simulink model "testEmplanner_cs_referencelinev01"  (R2021b)
settings: Solver=ode5  StartTime=0.0  StopTime=150  FixedStep=1/1000  RelTol=1e-3
PreLoadFcn:
  | mbxruntime.callbacks.PreLoadFcn(bdroot);
PostLoadFcn:
  | mbxruntime.callbacks.PostLoadFcn(bdroot);
InitFcn:
  | mbxruntime.callbacks.InitFcn(bdroot);
StartFcn:
  | mbxruntime.callbacks.StartFcn(bdroot);
StopFcn:
  | mbxruntime.callbacks.StopFcn(bdroot);
model workspace (MAT data in the model file):
  mbox_table : object (value not decoded)
  model_closed = 0
  sim_status = 0
values from neighbouring files (symbols this model uses):
  c_factor = 43.75    [emplanner_init.m]
  cf = -175016    [emplanner_init.m]
  cr = -130634    [emplanner_init.m]
  global_path_x = [-1.1448 -0.145417744933 0.852705365581 1.84955224935 2.84511712279 3.83939835808 4.83239585569 5.82411007764 6.81454169183 7.80369144113 8.79156009523 9.77814843293 ... (3001 elements, 3001x1)]    [global_path.mat]
  global_path_y = [14.6488 14.6488 14.6488 14.6488 14.6488 14.6488 14.6488 14.6488 14.6488 14.6488 14.6488 14.6488 ... (3001 elements, 3001x1)]    [global_path.mat]
  KD_PID_distance = 0.0    (= 0)    [emplanner_init.m]
  KD_PID_speed = 0    [emplanner_init.m]
  KI_PID_distance = 0.0    (= 0)    [emplanner_init.m]
  KI_PID_speed = 0    [emplanner_init.m]
  KP_PID_distance = 0.5    [emplanner_init.m]
  KP_PID_speed = 1.8    [emplanner_init.m]
  la = 1.265    [emplanner_init.m]
  lb = 2.947-1.265    (= 1.682)    [emplanner_init.m]
  LQR_K1 = k(:,1)'    [emplanner_init.m]
  LQR_K2 = k(:,2)'    [emplanner_init.m]
  LQR_K3 = k(:,3)'    [emplanner_init.m]
  LQR_K4 = k(:,4)'    [emplanner_init.m]
  m = 2020    [emplanner_init.m]
  rack_displacement = [-39.14 , -37.2 , -35.29 , -33.43 , -31.6 , -29.81 , -28.06 , -26.34 , -24.66 ,      -23.01 , -21.38 , -19.79 , -18.23 , -16.69 , -15.18 , -13.7 , -12.23 , -10.8 , -9.38 , -7.98 ,     -6.61 , -5.25 , -3.91 , -2.59 , -1.29 , 0 , 1.27 , 2.54 , 3.78 , 5.02 , 6.24 , 7.46 , 8.66 ,      9.86 , 11.05 , 12.24 , 13.41 , 14.59 , 15.76 , 16.92 , 18.09 , 19.25 , 20.42 , 21.59 , 22.76 ,      23.93 , 25.11 , 26 ...(+26 chars)    [emplanner_init.m]
  right_wheel_ground = [-70 ,-67.2 , -64.4 , -61.6 , -58.8 , -56 , -53.2 , -50.4 , -47.6 , -44.8 , -42 ,      -39.2 , -36.4 , -33.6 , -30.8 , -28 , -25.2 , -22.4 , -19.6 , -16.8 , -14 , -11.2 , -8.4 , -5.6 ,      -2.8 , 0 , 2.8 , 5.6 , 8.4 , 11.2 , 14 , 16.8 , 19.6 , 22.4 , 25.2 , 28 , 30.8 , 33.6 , 36.4 ,      39.2 , 42 , 44.8 , 47.6 , 50.4 , 53.2 , 56 , 58.8 , 61.6 , 64.4 , 67.2 , 70 ]    [emplanner_init.m]
  vx_break_point = zeros(1,5000)    [emplanner_init.m]
undefined symbols (not defined in the file or in its folder): aubr, DiscIntNeverNeededParam, tablebr, vubr, warningInitialVelocity, x0
libraries: simulink x19, PreScanSimulinkLibrary x9, simulink_extras x6, Solver_SF x1
(part 5 of 5)

== system testEmplanner_cs_referencelinev01/Audi_A8_Sedan_2/Dynamics_Simple/Chassis/Bicycle_model_[XYZ]/Z, Pitch_Motion & Roll_Motion/Configurable Subsystem1 ==
  In1 : Inport
  Integrator : Integrator
  Out1 : Outport
  wires:
  In1/1 -> Integrator/1
  Integrator/1 -> Out1/1

== system testEmplanner_cs_referencelinev01/Audi_A8_Sedan_2/Dynamics_Simple/Chassis/Bicycle_model_[XYZ]/Z, Pitch_Motion & Roll_Motion/Configurable Subsystem2 ==
  In1 : Inport
  Integrator : Integrator
  Out1 : Outport
  wires:
  In1/1 -> Integrator/1
  Integrator/1 -> Out1/1

== system testEmplanner_cs_referencelinev01/Audi_A8_Sedan_2/Dynamics_Simple/Chassis/Bicycle_model_[XYZ]/Z, Pitch_Motion & Roll_Motion/Configurable Subsystem3 ==
  In1 : Inport
  Integrator : Integrator
  Out1 : Outport
  wires:
  In1/1 -> Integrator/1
  Integrator/1 -> Out1/1

== system testEmplanner_cs_referencelinev01/Audi_A8_Sedan_2/Dynamics_Simple/Chassis/Bicycle_model_[XYZ]/Z, Pitch_Motion & Roll_Motion/Configurable Subsystem4 ==
  In1 : Inport
  Integrator : Integrator
  Out1 : Outport
  wires:
  In1/1 -> Integrator/1
  Integrator/1 -> Out1/1

== system testEmplanner_cs_referencelinev01/Audi_A8_Sedan_2/Dynamics_Simple/Chassis/Bicycle_model_[XYZ]/Z, Pitch_Motion & Roll_Motion/Configurable Subsystem5 ==
  In1 : Inport
  Integrator : Integrator
  Out1 : Outport
  wires:
  In1/1 -> Integrator/1
  Integrator/1 -> Out1/1

== system testEmplanner_cs_referencelinev01/Audi_A8_Sedan_2/Dynamics_Simple/Chassis/Bicycle_model_[XYZ]/Z, Pitch_Motion & Roll_Motion/Configurable Subsystem9 ==
  In1 : Inport
  Derivative : Derivative
  Out1 : Outport
  wires:
  In1/1 -> Derivative/1
  Derivative/1 -> Out1/1

== system testEmplanner_cs_referencelinev01/Audi_A8_Sedan_2/Dynamics_Simple/Chassis/FrontTyre/AlphaFront/Enabled Subsystem ==
  In : Inport
  Enable : EnablePort  PropagateVarSize=During execution
  AlphaFront : Fcn  Expr=-atan( (u(2)+u(3)*p.a)/u(1) )
  Alpha : Outport  OutputWhenDisabled=reset  InitialOutput=[0]
  wires:
  AlphaFront/1 -> Alpha/1
  In/1 -> AlphaFront/1

== system testEmplanner_cs_referencelinev01/Audi_A8_Sedan_2/Dynamics_Simple/Chassis/RearTyre/AlphaRear/Enabled Subsystem ==
  In : Inport
  Enable : EnablePort  PropagateVarSize=During execution
  AlphaRear : Fcn  Expr=-atan( (u(2)-u(3)*p.b)/u(1) )
  Alpha : Outport  OutputWhenDisabled=reset  InitialOutput=[0]
  wires:
  AlphaRear/1 -> Alpha/1
  In/1 -> AlphaRear/1

== system testEmplanner_cs_referencelinev01/Audi_A8_Sedan_2/Trajectories/Traj2State1/Traj2State2/Traj2MuxState_Ext/demux ==
  traj : Inport
  Demux : Demux  Outputs=18
  x : Outport
  y : Outport  Port=2
  z : Outport  Port=3
  velx : Outport  Port=4
  vely : Outport  Port=5
  velz : Outport  Port=6
  R : Outport  Port=7
  P : Outport  Port=8
  Y : Outport  Port=9
  velR : Outport  Port=10
  velP : Outport  Port=11
  velY : Outport  Port=12
  accx : Outport  Port=13
  accy : Outport  Port=14
  accz : Outport  Port=15
  accR : Outport  Port=16
  accP : Outport  Port=17
  accY : Outport  Port=18
  wires:
  Demux/18 -> accY/1
  Demux/17 -> accP/1
  Demux/16 -> accR/1
  Demux/15 -> accz/1
  Demux/14 -> accy/1
  Demux/13 -> accx/1
  Demux/12 -> velY/1
  Demux/11 -> velP/1
  Demux/10 -> velR/1
  Demux/9 -> velz/1
  Demux/8 -> vely/1
  Demux/7 -> velx/1
  Demux/6 -> Y/1
  Demux/5 -> P/1
  traj/1 -> Demux/1
  Demux/4 -> R/1
  Demux/3 -> z/1
  Demux/2 -> y/1
  Demux/1 -> x/1

== system testEmplanner_cs_referencelinev01/Audi_A8_Sedan_2/Dynamics_Simple/Chassis/Bicycle_model_[XYZ]/X_Motion/Max RPM and zero- velocity detection/Configurable Subsystem ==
  Step : Step  Time=0.0001  Before=1  After=0  SampleTime=0
  Out1 : Outport
  wires:
  Step/1 -> Out1/1

== system testEmplanner_cs_referencelinev01/Audi_A8_Sedan_2/Dynamics_Simple/Chassis/Bicycle_model_[XYZ]/X_Motion/Max RPM and zero- velocity detection/SR-Memory ==
  Signal : Inport
  Set : Inport  Port=2
  Reset : Inport  Port=3
  Constant : Constant  Value=0
  Detect Rise Positive : simulink/Logic and Bit Operations/Detect Rise Positive  vinit=0  OutDataTypeStr=uint8
  Detect Rise Positive1 : simulink/Logic and Bit Operations/Detect Rise Positive  vinit=0  OutDataTypeStr=uint8
  Manual Switch : ManualSwitch
  Manual Switch1 : ManualSwitch
  Switch : Switch  Criteria=u2 ~= 0
  Switch1 : Switch  Criteria=u2 ~= 0
  Unit Delay : UnitDelay  SampleTime=-1  HasFrameUpgradeWarning=on
  Out : Outport
  wires:
  Constant/1 -> Switch1/1
  Switch/1 -> Switch1/3
  Switch1/1 -> Unit Delay/1, Out/1
  Manual Switch1/1 -> Switch1/2
  Reset/1 -> Manual Switch1/2, Detect Rise Positive1/1
  Detect Rise Positive1/1 -> Manual Switch1/1
  Signal/1 -> Switch/1
  Unit Delay/1 -> Switch/3
  Set/1 -> Detect Rise Positive/1, Manual Switch/2
  Detect Rise Positive/1 -> Manual Switch/1
  Manual Switch/1 -> Switch/2

== matlab function testEmplanner_cs_referencelinev01/Audi_A8_Sedan_1/decision&planning module/referenceline provider/MATLAB Function ==
  data: x_set input; match_point_index_set output; y_set input; frenet_path_x input; frenet_path_y input; frenet_path_heading input; frenet_path_kappa input; proj_x_set output; proj_y_set output; proj_heading_set output; proj_kappa_set output
function [match_point_index_set,proj_x_set,proj_y_set,proj_heading_set,proj_kappa_set] = ...
	fcn(x_set,y_set,frenet_path_x,frenet_path_y,frenet_path_heading,frenet_path_kappa)
	
%该函数将批量计算x_set,y_set中(x,y) 在frenet坐标系下的投影信息
%输入： x_set，y_set 待投影的点的集合
	%x_set,y_set,frenet_path_x,frenet_path_y,frenet_path_heading,frenet_path_kappa
	%曲线在直角坐标系下的x,y,heading,kappa
%输出：math_point_index_set 匹配点在frenet_path下的编号的集合（即从全局路径的第一个点开始数，第几个点是匹配点）

%由于事先不知道x_set中有多少个点需要投影，因此事先声明一个最大数量的点作为缓冲

n = 128;
%并且不知道投影点的数量，所以也不知道输出的数量，因此输出也要做缓冲，用nan表示不存在的点
%初始化输出最多为128个点。
%输出初始化
match_point_index_set = ones(n,1) * nan;
proj_x_set = ones(n,1) * nan;
proj_y_set = ones(n,1) * nan;
proj_heading_set = ones(n,1) * nan;
proj_kappa_set = ones(n,1) * nan;

%找匹配点，需要利用上一个周期的结果作为下一个周期遍历的起点，因此需要声明两个全局变量
persistent is_first_run;
persistent pre_match_point_index_set;
persistent pre_frenet_path_x;
persistent pre_frenet_path_y;
persistent pre_frenet_path_heading;
persistent pre_frenet_path_kappa;

%算法主函数入口

if isempty(is_first_run)
	% 该if分支表示函数首次运行
	is_first_run = 0; %赋值
	pre_frenet_path_x = frenet_path_x;
	pre_frenet_path_y = frenet_path_y;
	pre_frenet_path_heading = frenet_path_heading;
	pre_frenet_path_kappa = frenet_path_kappa;
	%记录首次运行计算的匹配点的结果供下个周期运行，先初始化
	pre_match_point_index_set = ones(n,1) * nan;
	
	%对x_set,y_set的点做遍历，找到他们的匹配点
	for i = 1 : length(x_set)
		%首次运行时，没有任何提示，只能从frenet_path的第一个点开始找
		start_search_index = 1;
		%声明increa_count,用于表示在遍历时distance连续增大的次数
		increase_count = 0;
		%开始遍历
		min_distance = inf;
		for j = start_search_index : length(frenet_path_x)
			distance = (x_set(i) - frenet_path_x(j))^2 + (y_set(i) - frenet_path_y(j))^2;
			%处理最小值
			if distance < min_distance
				min_distance = distance;
				match_point_index_set(i) = j; %math_point_index_set存放匹配点的序号
				increase_count = 0;
			else
				increase_count = increase_count + 1;
			end
			% 如果连续distanc增加50次,就不要再遍历了，节省时间
			if increase_count > 50 
				break;
			end	
		end
		%如何通过匹配点计算投影点，参考《自动驾驾驶控制算法第七讲》
		%或者《自动驾驶决策规划算法》第一章第三节
		
		%取出匹配点的编号
		match_point_index = match_point_index_set(i);
		
		%取出匹配点信息
		match_point_x = frenet_path_x(match_point_index);
		match_point_y = frenet_path_y(match_point_index);
		match_point_heading = frenet_path_heading(match_point_index);
		match_point_kappa = frenet_path_kappa(match_point_index);
		
		% 计算匹配点的位置向量和方向向量
		vector_match_point = [match_point_x;match_point_y];%位置向量
		vector_match_point_direction = [cos(match_point_heading);sin(match_point_heading)];%方向向量，全局坐标系下（大地坐标系）
		
		%声明待投影点的位矢
		vector_r = [x_set(i);y_set(i)];
		
		%通过匹配点计算投影点
		vector_d = vector_r - vector_match_point;
		ds = vector_d' * vector_match_point_direction;
		vector_proj_point = vector_match_point + vector_match_point_direction *ds;
		proj_heading = match_point_heading + match_point_kappa * ds;
		proj_kappa = match_point_kappa;
		
		%计算结果输出 
		proj_x_set(i) = vector_proj_point(1);
		proj_y_set(i) = vector_proj_point(2);
		proj_heading_set(i) = proj_heading;
		proj_kappa_set(i) = proj_kappa;
	end
	
	%匹配点的计算结果保存，供下一个周期使用
	pre_match_point_index_set = match_point_index_set;
else
	% 此分支不是首次运行
	
	%对每个x_set上的点做处理
	for i = 1 : length(x_set)
		%不是首次运行，对于点x_set(i),y_set(i)来说，start_search_index = pre_match_point_index_set(i)
		start_search_index = pre_match_point_index_set(i);%上个周期匹配点的编号作为本周期搜索的起点
		
		%声明increa_count,用于表示在遍历时distance连续增大的次数
		increase_count = 0;
		%开始遍历
		
		%这里多了一个步骤，判断遍历的方向
		%计算上个周期匹配点的位失
		vector_pre_match_point = [pre_frenet_path_x(start_search_index); pre_frenet_path_y(start_search_index)];
		vector_pre_match_point_direction = ...
			[cos(pre_frenet_path_heading(start_search_index));sin(pre_frenet_path_heading(start_search_index))];
		
		% 判断遍历的方向
		flag = ([x_set(i);y_set(i)] - vector_pre_match_point)' * vector_pre_match_point_direction;
		
		min_distance = inf;
		
		if flag > 0.001 
			for j = start_search_index : length(frenet_path_x)
				distance = (x_set(i) - frenet_path_x(j))^2 + (y_set(i) - frenet_path_y(j))^2;
				%处理最小值
				if distance < min_distance
					min_distance = distance;
					match_point_index_set(i) = j; %math_point_index_set存放匹配点的序号
					increase_count = 0;
				else
					increase_count = increase_count + 1;
				end
				% 如果连续distanc增加5次,就不要再遍历了，节省时间
				if increase_count > 5 
					break;
				end
			end
		elseif flag < -0.001
			for j = start_search_index :-1: 1
				distance = (x_set(i) - frenet_path_x(j))^2 + (y_set(i) - frenet_path_y(j))^2;
				%处理最小值
				if distance < min_distance
					min_distance = distance;
					match_point_index_set(i) = j; %math_point_index_set存放匹配点的序号
					increase_count = 0;
				else
					increase_count = increase_count + 1;
				end
				% 如果连续distanc增加50次,就不要再遍历了，节省时间
				if increase_count > 5 
					break;
				end
			end
		else
			match_point_index_set(i) = start_search_index;
		end
			
		%如何通过匹配点计算投影点，参考《自动驾驾驶控制算法第七讲》
		%或者《自动驾驶决策规划算法》第一章第三节
		
		%取出匹配点的编号
		match_point_index = match_point_index_set(i);
		
		%取出匹配点信息
		match_point_x = frenet_path_x(match_point_index);
		match_point_y = frenet_path_y(match_point_index);
		match_point_heading = frenet_path_heading(match_point_index);
		match_point_kappa = frenet_path_kappa(match_point_index);
		
		% 计算匹配点的位置向量和方向向量
		vector_match_point = [match_point_x;match_point_y];%位置向量
		vector_match_point_direction = [cos(match_point_heading);sin(match_point_heading)];%方向向量
		
		%声明待投影点的位矢
		vector_r = [x_set(i);y_set(i)];
		
		%通过匹配点计算投影点
		vector_d = vector_r - vector_match_point;
		ds = vector_d' * vector_match_point_direction;
		vector_proj_point = vector_match_point + ds * vector_match_point_direction;
		proj_heading = match_point_heading + match_point_kappa * ds;
		proj_kappa = match_point_kappa;
		
		%计算结果输出 
		proj_x_set(i) = vector_proj_point(1);
		proj_y_set(i) = vector_proj_point(2);
		proj_heading_set(i) = proj_heading;
		proj_kappa_set(i) = proj_kappa;
	end
	
	%匹配点的计算结果保存，供下一个周期使用
	pre_match_point_index_set = match_point_index_set;
	pre_frenet_path_x = frenet_path_x;
	pre_frenet_path_y = frenet_path_y;
	pre_frenet_path_heading = frenet_path_heading;
	pre_frenet_path_kappa = frenet_path_kappa;
end

== matlab function testEmplanner_cs_referencelinev01/Audi_A8_Sedan_1/decision&planning module/referenceline provider/MATLAB Function1 ==
  data: path_x input; path_heading output; path_y input; path_kappa output
function [path_heading,path_kappa] = fcn(path_x,path_y)
%该函数将计算path的切线方向与x轴的夹角和曲率
%输入：path_x,path_y路径的坐标（全局坐标系下）
%输出：path_heading,path_kappa 路径的heading和曲率
%原理：heading = arctan(dy/dx)
%  kappa = dheading /ds
%  ds = (dx^2 + dy^2)^0.5


%注意，角度的多值性会带来很大的麻烦，需要慎重处理
%例如： x与 x+2*pi代表同一个角度，这种多值性在曲率计算的时候会带来麻烦
%比如： 原本是（0.1 -（-0.1））/ ds,但是如果计算出得-0.1多了一个2*pi
%kappa 就等于(0.1 -(-0.1 + 2*pi)) /ds 曲率就会变得非常大
%还有若采用中点欧拉法计算heading时，即使用 (y2 - y1) / (x2 - x1)的反正切计算一个角度，用(y1 - y0)/(x1 - x0)的反正切
%又计算了一个角度，然后加起来除以2，如果精确值是(a1 + a2)/2,但是最终计算结果可能是(a1 + a2 + 2pi) / 2
%还有tan(x) = tan(x + pi） 所以 arctan(tan(x)) 可能等于x,也可能等于x + pi
%角度的处理非常麻烦，而且角度处理不当往往是许多奇怪错误的源头
%

dx = diff(path_x);
dy = diff(path_y);%计算差分

%用中点欧拉法要比向前欧拉法和向后欧拉法要更精确，但是也可能计算出的结果比精确值多一个pi
%在这里对dx,dy做中点欧拉法，使用四象限反正切计算角度

dx_pre = [dx(1);dx];
dx_after = [dx;dx(end)];
dx_final = (dx_pre + dx_after) / 2;

dy_pre = [dy(1);dy];
dy_after = [dy;dy(end)];
dy_final = (dy_pre + dy_after) / 2;

ds_final = sqrt(dx_final.^2 + dy_final.^2);
path_heading = atan2(dy_final,dx_final);

%atan2(b，a)：4象限反正切，

%　　　　计算b/a对应的反正切值，求点(a，b)对应的角
% 　　　　　(a，b)位于第一象限时，atan2(b，a)取值  0 ~ pi/2
% 　　　　　(a，b)位于第二象限时，atan2(b，a)取值  pi/2 ~ pi
% 　　　　　(a，b)位于第三象限时，atan2(b，a)取值   -pi ~ -pi/2
% 　　　　　(a，b)位于第四象限时，atan2(b，a)取值   -pi/2 ~ 0
%

%中点欧拉法
dheading = diff(path_heading);%差分，size变成length(path_heading) - 1
dheading_pre = [dheading(1);dheading]; %插入一个首元素
dheading_after = [dheading;dheading(end)]; %插入一个尾元素
dheading_final = (dheading_pre + dheading_after) / 2;
%为了防止dheading出现一个2*pi的错误，假设真实的heading较小，用sin(dheading)近似dheading
path_kappa = sin(dheading_final)./ds_final;

== matlab function testEmplanner_cs_referencelinev01/Audi_A8_Sedan_2/PathFollower_Preview_1/LateralController/Calculate delta steering error/eml_delta_steering_error ==
  data: v_x_vehicle input; v_x_vehicle_Min input; t_Preview_LatCtrl input; delta_steeringwheeltotal output; v_y_vehicle input; yawrate_vehicle input; CorneringStiffness_Tyres_Front input; CorneringStiffness_Tyres_Rear input; m_vehicle_total input; inertia_z_vehicle_total input; e_Lat input size=10; Pos_x_CoG_Vehicle input; wheelbase input; RefreshCounter parameter
function delta_steeringwheeltotal = eml_delta_steering_error(v_x_vehicle,v_x_vehicle_Min,t_Preview_LatCtrl,v_y_vehicle,yawrate_vehicle,CorneringStiffness_Tyres_Front,CorneringStiffness_Tyres_Rear,m_vehicle_total,inertia_z_vehicle_total,e_Lat,Pos_x_CoG_Vehicle,wheelbase,RefreshCounter)

delta_steeringwheeltotal = emlfcn_delta_steering_error(v_x_vehicle,v_x_vehicle_Min,t_Preview_LatCtrl,v_y_vehicle,yawrate_vehicle,CorneringStiffness_Tyres_Front,CorneringStiffness_Tyres_Rear,m_vehicle_total,inertia_z_vehicle_total,e_Lat,Pos_x_CoG_Vehicle,wheelbase,RefreshCounter);

% end function

== matlab function testEmplanner_cs_referencelinev01/Audi_A8_Sedan_1/decision&planning module/referenceline provider/MATLAB Function3 ==
  data: match_point_index_set input; match_point_index output
function match_point_index = fcn(match_point_index_set)
match_point_index = match_point_index_set(1);

== matlab function testEmplanner_cs_referencelinev01/Audi_A8_Sedan_1/decision&planning module/referenceline provider/MATLAB Function4 ==
  data: referenceline_x_init input; referenceline_x output; referenceline_y_init input; w_cost_smooth input; w_cost_length input; w_cost_ref input; x_lb input; x_ub input; y_lb input; y_ub input; referenceline_y output
function [referenceline_x,referenceline_y] = ...
 	fcn(referenceline_x_init,referenceline_y_init,w_cost_smooth,w_cost_length,w_cost_ref,x_lb,x_ub,y_lb,y_ub)
 %该函数将平滑referenceline
 %使用二次规划算法
 %原理：
 %	0.5x'Hx + f'x = min 
 %约束条件:
 %	lb <= x <= ub
 %输入： referenceline_x_init,referenceline_y_init,未平滑的参考线
 %w_cost_smooth,w_cost_length,w_cost_ref 平滑代价，紧凑代价，几何相似代价权重系数
 %x_lb,x_ub,y_lb,y_ub 允许x,y变化的上下界
 %输出：referenceline_x,referenceline_y 平滑后的参考线
 
 %这里为了简化，不适用拼接算法
 %计算量问题通过调度器来解决，规划周期设置100ms，只要在100ms完成就可以了
 %如果到最后计算速度还是问题，再进行优化，目前暂时不适用拼接算法
 
 %simulink 无法直接使用自带的二次规划函数，需要从外部引入，执行下面命令
 
 coder.extrinsic("quadprog");
  %二次规划的形式
%   H1 = w_cost_smooth * (A1'*A1) + w_cost_length*(A2'*A2) + w_cost_ref * (A3'*A3)
%   f = -2 * w_cost_ref * referenceline_x 
%   x’H1x + f'x = 0.5 * x'(2H1)*x + f'x
%   A1 = [1 0 -2 0 1 0 
%            1 0 -2 0 1 
%              1  0 -2 0 1 
%                    .........
%  
%   A2 = [ 1 0 -1 0
%            1 0  -1 0 
%              1 0 -1 0
%                1 0  -1 0 
%                  ........
 
 %A3 为单位矩阵
 
 %设置求解矩阵的规模，因为参考线初始点一共181个，每个点有两个坐标，所以求解矩阵规模是362
 n = 181;
 %referenceline初始化
 referenceline_x = zeros(n,1);
 referenceline_y = zeros(n,1);
 
 
 A1 = zeros(2 * n - 4, 2 * n);
 A2 = zeros(2 * n - 2, 2 * n);
 A3 = eye(2 * n,2 * n);
 f = zeros(2 * n,1);
 lb = zeros(2 * n,1);
 ub = zeros(2 * n,1);
 persistent is_first_run;
 persistent pre_result_x;
 persistent pre_result_y;
 persistent pre_referenceline_x_init;
 persistent pre_referenceline_y_init;
 
 if isempty(is_first_run)
 	is_first_run = 0;
 	% 一个坐标具有两个值,f(2*i-1)是对应的x,f(2*i)是对应的y
 	for i = 1 : n
 		f(2*i - 1) = referenceline_x_init(i);
 		f(2*i) = referenceline_y_init(i);
 		lb(2*i-1) = f(2*i - 1) + x_lb;
 		ub(2*i-1) = f(2*i - 1) + x_ub;
 		lb(2*i) = f(2*i) + y_lb;
 		ub(2*i) = f(2*i) + y_ub;
 	end
 
 	for j = 1 : 2 : 2 * n - 5
 		A1(j,j) = 1;
 		A1(j,j+2) = -2;
 		A1(j,j+4) = 1;
 		A1(j+1,j+1) = 1;
 		A1(j+1,j+3) = -2;
 		A1(j+1,j+5) = 1;
 	end
 
 	for k = 1 : 2 :2 * n -3
 		A2(k,k) = 1;
 		A2(k,k+2) = -1;
 		A2(k+1,k+1) = 1;
 		A2(k+1,k+3) = -1;
 	end
 
 	H1 = w_cost_smooth * (A1'*A1)  + w_cost_length *(A2'*A2) + w_cost_ref * A3;
 	H = 2 * H1;
 	%用 referenceline的初值作为二次规划的迭代的起点,加速二次规划的过程
 	X0 = f;
 	f = -2 * w_cost_ref * f;
 	
 	%二次规划求解
 	X = quadprog(H,f,[],[],[],[],lb,ub,X0);
 	%将结果输出到referenceline中
 	for i = 1 : n 
 		referenceline_x(i) = X(2*i -1);
 		referenceline_y(i) = X(2*i);
 	end
 	pre_result_x = referenceline_x;
 	pre_result_y = referenceline_y;
 	pre_referenceline_x_init = referenceline_x_init;
 	pre_referenceline_y_init = referenceline_y_init;
 else
    if pre_referenceline_x_init(1) == referenceline_x_init(1) && ...
 		pre_referenceline_y_init(1) == referenceline_y_init(1) 
 		 %起点相同，可以认为本周期和上个周期reference_init 完全相同，直接使用
 		referenceline_x = pre_result_x;
 		referenceline_y = pre_result_y;
    else
        for i = 1 : n
 			f(2*i - 1) = referenceline_x_init(i);
 			f(2*i) = referenceline_y_init(i);
 			lb(2*i-1) = f(2*i - 1) + x_lb;
 			ub(2*i-1) = f(2*i - 1) + x_ub;
 			lb(2*i) = f(2*i) + y_lb;
 			ub(2*i) = f(2*i) + y_ub;
        end
 
 		for j = 1 : 2 : 2 * n - 5
 			A1(j,j) = 1;
 			A1(j,j+2) = -2;
 			A1(j,j+4) = 1;
 			A1(j+1,j+1) = 1;
 			A1(j+1,j+3) = -2;
 			A1(j+1,j+5) = 1;
 		end
 
        for k = 1 : 2 : 2*n -3
 			A2(k,k) = 1;
 			A2(k,k+2) = -1;
 			A2(k+1,k+1) = 1;
 			A2(k+1,k+3) = -1;
        end 	
 	    H1 = w_cost_smooth * (A1'*A1)  + w_cost_length *(A2'*A2) + w_cost_ref * A3;
 	    H = 2 * H1;
 	    %用 referenceline的初值作为二次规划的迭代的起点,加速二次规划的过程
 	    X0 = f ;
 	    f = -2 * w_cost_ref * f;
 	    
 	    %二次规划求解
 	    X = quadprog(H,f,[],[],[],[],lb,ub,X0);
 	    %将结果输出到referenceline中
 	    for i = 1 :n 
 		    referenceline_x(i) = X(2*i -1);
 		    referenceline_y(i) = X(2*i);
 	    end
 	    pre_result_x = referenceline_x;
 	    pre_result_y = referenceline_y;
 	    pre_referenceline_x_init = referenceline_x_init;
 	    pre_referenceline_y_init = referenceline_y_init;
    end
 end

== matlab function testEmplanner_cs_referencelinev01/Audi_A8_Sedan_1/decision&planning module/MATLAB Function ==
  data: x_set input; match_point_index_set output; y_set input; frenet_path_x input; frenet_path_y input; frenet_path_heading input; frenet_path_kappa input; proj_x_set output; proj_y_set output; proj_heading_set output; proj_kappa_set output
function [match_point_index_set,proj_x_set,proj_y_set,proj_heading_set,proj_kappa_set] = ...
	fcn(x_set,y_set,frenet_path_x,frenet_path_y,frenet_path_heading,frenet_path_kappa)
	
%该函数将批量计算x_set,y_set中(x,y) 在frenet坐标系下的投影信息
%输入： x_set，y_set 待投影的点的集合
	%x_set,y_set,frenet_path_x,frenet_path_y,frenet_path_heading,frenet_path_kappa
	%曲线在直角坐标系下的x,y,heading,kappa
%输出：math_point_index_set 匹配点在frenet_path下的编号的集合（即从全局路径的第一个点开始数，第几个点是匹配点）

%由于事先不知道x_set中有多少个点需要投影，因此事先声明一个最大数量的点作为缓冲

n = 128;
%并且不知道投影点的数量，所以也不知道输出的数量，因此输出也要做缓冲，用nan表示不存在的点
%初始化输出最多为128个点。
%输出初始化
match_point_index_set = ones(n,1) * nan;
proj_x_set = ones(n,1) * nan;
proj_y_set = ones(n,1) * nan;
proj_heading_set = ones(n,1) * nan;
proj_kappa_set = ones(n,1) * nan;

%找匹配点，需要利用上一个周期的结果作为下一个周期遍历的起点，因此需要声明两个全局变量
persistent is_first_run;
persistent pre_match_point_index_set;
persistent pre_frenet_path_x;
persistent pre_frenet_path_y;
persistent pre_frenet_path_heading;
persistent pre_frenet_path_kappa;

%算法主函数入口

if isempty(is_first_run)
	% 该if分支表示函数首次运行
	is_first_run = 0; %赋值
	pre_frenet_path_x = frenet_path_x;
	pre_frenet_path_y = frenet_path_y;
	pre_frenet_path_heading = frenet_path_heading;
	pre_frenet_path_kappa = frenet_path_kappa;
	%记录首次运行计算的匹配点的结果供下个周期运行，先初始化
	pre_match_point_index_set = ones(n,1) * nan;
	
	%对x_set,y_set的点做遍历，找到他们的匹配点
	for i = 1 : length(x_set)
		%首次运行时，没有任何提示，只能从frenet_path的第一个点开始找
		start_search_index = 1;
		%声明increa_count,用于表示在遍历时distance连续增大的次数
		increase_count = 0;
		%开始遍历
		min_distance = inf;
		for j = start_search_index : length(frenet_path_x)
			distance = (x_set(i) - frenet_path_x(j))^2 + (y_set(i) - frenet_path_y(j))^2;
			%处理最小值
			if distance < min_distance
				min_distance = distance;
				match_point_index_set(i) = j; %math_point_index_set存放匹配点的序号
				increase_count = 0;
			else
				increase_count = increase_count + 1;
			end
			% 如果连续distanc增加50次,就不要再遍历了，节省时间
			if increase_count > 50 
				break;
			end	
		end
		%如何通过匹配点计算投影点，参考《自动驾驾驶控制算法第七讲》
		%或者《自动驾驶决策规划算法》第一章第三节
		
		%取出匹配点的编号
		match_point_index = match_point_index_set(i);
		
		%取出匹配点信息
		match_point_x = frenet_path_x(match_point_index);
		match_point_y = frenet_path_y(match_point_index);
		match_point_heading = frenet_path_heading(match_point_index);
		match_point_kappa = frenet_path_kappa(match_point_index);
		
		% 计算匹配点的位置向量和方向向量
		vector_match_point = [match_point_x;match_point_y];%位置向量
		vector_match_point_direction = [cos(match_point_heading);sin(match_point_heading)];%方向向量，全局坐标系下（大地坐标系）
		
		%声明待投影点的位矢
		vector_r = [x_set(i);y_set(i)];
		
		%通过匹配点计算投影点
		vector_d = vector_r - vector_match_point;
		ds = vector_d' * vector_match_point_direction;
		vector_proj_point = vector_match_point + ds * vector_match_point_direction;
		proj_heading = match_point_heading + match_point_kappa * ds;
		proj_kappa = match_point_kappa;
		
		%计算结果输出 
		proj_x_set(i) = vector_proj_point(1);
		proj_y_set(i) = vector_proj_point(2);
		proj_heading_set(i) = proj_heading;
		proj_kappa_set(i) = proj_kappa;
	end
	
	%匹配点的计算结果保存，供下一个周期使用
	pre_match_point_index_set = match_point_index_set;
else
	% 此分支不是首次运行
	
	%对每个x_set上的点做处理
	for i = 1 : length(x_set)
		%不是首次运行，对于点x_set(i),y_set(i)来说，start_search_index = pre_match_point_index_set(i)
		start_search_index = pre_match_point_index_set(i);%上个周期匹配点的编号作为本周期搜索的起点
		
		%声明increa_count,用于表示在遍历时distance连续增大的次数
		increase_count = 0;
		%开始遍历
		
		%这里多了一个步骤，判断遍历的方向
		%计算上个周期匹配点的位失
		vector_pre_match_point = [pre_frenet_path_x(start_search_index); pre_frenet_path_y(start_search_index)];
		vector_pre_match_point_direction = ...
			[cos(pre_frenet_path_heading(start_search_index));sin(pre_frenet_path_heading(start_search_index))];
		
		% 判断遍历的方向
		flag = ([x_set(i);y_set(i)] - vector_pre_match_point)' * vector_pre_match_point_direction;
		
		min_distance = inf;
		
		if flag > 0.001 
			for j = start_search_index : length(frenet_path_x)
				distance = (x_set(i) - frenet_path_x(j))^2 + (y_set(i) - frenet_path_y(j))^2;
				%处理最小值
				if distance < min_distance
					min_distance = distance;
					match_point_index_set(i) = j; %math_point_index_set存放匹配点的序号
					increase_count = 0;
				else
					increase_count = increase_count + 1;
				end
				% 如果连续distanc增加5次,就不要再遍历了，节省时间
				if increase_count > 5 
					break;
				end
			end
		elseif flag < -0.001
			for j = start_search_index :-1: 1
				distance = (x_set(i) - frenet_path_x(j))^2 + (y_set(i) - frenet_path_y(j))^2;
				%处理最小值
				if distance < min_distance
					min_distance = distance;
					match_point_index_set(i) = j; %math_point_index_set存放匹配点的序号
					increase_count = 0;
				else
					increase_count = increase_count + 1;
				end
				% 如果连续distanc增加50次,就不要再遍历了，节省时间
				if increase_count > 5 
					break;
				end
			end
		else
			match_point_index_set(i) = start_search_index;
		end
			
		%如何通过匹配点计算投影点，参考《自动驾驾驶控制算法第七讲》
		%或者《自动驾驶决策规划算法》第一章第三节
		
		%取出匹配点的编号
		match_point_index = match_point_index_set(i);
		
		%取出匹配点信息
		match_point_x = frenet_path_x(match_point_index);
		match_point_y = frenet_path_y(match_point_index);
		match_point_heading = frenet_path_heading(match_point_index);
		match_point_kappa = frenet_path_kappa(match_point_index);
		
		% 计算匹配点的位置向量和方向向量
		vector_match_point = [match_point_x;match_point_y];%位置向量
		vector_match_point_direction = [cos(match_point_heading);sin(match_point_heading)];%方向向量
		
		%声明待投影点的位矢
		vector_r = [x_set(i);y_set(i)];
		
		%通过匹配点计算投影点
		vector_d = vector_r - vector_match_point;
		ds = vector_d' * vector_match_point_direction;
		vector_proj_point = vector_match_point + ds * vector_match_point_direction;
		proj_heading = match_point_heading + match_point_kappa * ds;
		proj_kappa = match_point_kappa;
		
		%计算结果输出 
		proj_x_set(i) = vector_proj_point(1);
		proj_y_set(i) = vector_proj_point(2);
		proj_heading_set(i) = proj_heading;
		proj_kappa_set(i) = proj_kappa;
	end
	
	%匹配点的计算结果保存，供下一个周期使用
	pre_match_point_index_set = match_point_index_set;
	pre_frenet_path_x = frenet_path_x;
	pre_frenet_path_y = frenet_path_y;
	pre_frenet_path_heading = frenet_path_heading;
	pre_frenet_path_kappa = frenet_path_kappa;
end

== matlab function testEmplanner_cs_referencelinev01/Audi_A8_Sedan_1/decision&planning module/MATLAB Function1 ==
  data: path_x input; path_heading output; path_y input; path_kappa output
function [path_heading,path_kappa] = fcn(path_x,path_y)
%该函数将计算path的切线方向与x轴的夹角和曲率
%输入：path_x,path_y路径的坐标（全局坐标系下）
%输出：path_heading,path_kappa 路径的heading和曲率
%原理：heading = arctan(dy/dx)
%  kappa = dheading /ds
%  ds = (dx^2 + dy^2)^0.5


%注意，角度的多值性会带来很大的麻烦，需要慎重处理
%例如： x与 x+2*pi代表同一个角度，这种多值性在曲率计算的时候会带来麻烦
%比如： 原本是（0.1 -（-0.1））/ ds,但是如果计算出得-0.1多了一个2*pi
%kappa 就等于(0.1 -(-0.1 + 2*pi)) /ds 曲率就会变得非常大
%还有若采用中点欧拉法计算heading时，即使用 (y2 - y1) / (x2 - x1)的反正切计算一个角度，用(y1 - y0)/(x1 - x0)的反正切
%又计算了一个角度，然后加起来除以2，如果精确值是(a1 + a2)/2,但是最终计算结果可能是(a1 + a2 + 2pi) / 2
%还有tan(x) = tan(x + pi） 所以 arctan(tan(x)) 可能等于x,也可能等于x + pi
%角度的处理非常麻烦，而且角度处理不当往往是许多奇怪错误的源头
%

dx = diff(path_x);
dy = diff(path_y);%计算差分

%用中点欧拉法要比向前欧拉法和向后欧拉法要更精确，但是也可能计算出的结果比精确值多一个pi
%在这里对dx,dy做中点欧拉法，使用四象限反正切计算角度

dx_pre = [dx(1);dx];
dx_after = [dx;dx(end)];
dx_final = (dx_pre + dx_after) / 2;

dy_pre = [dy(1);dy];
dy_after = [dy;dy(end)];
dy_final = (dy_pre + dy_after) / 2;

ds_final = sqrt(dx_final.^2 + dy_final.^2);
path_heading = atan2(dy_final,dx_final);

%atan2(b，a)：4象限反正切，

%　　　　计算b/a对应的反正切值，求点(a，b)对应的角
% 　　　　　(a，b)位于第一象限时，atan2(b，a)取值  0 ~ pi/2
% 　　　　　(a，b)位于第二象限时，atan2(b，a)取值  pi/2 ~ pi
% 　　　　　(a，b)位于第三象限时，atan2(b，a)取值   -pi ~ -pi/2
% 　　　　　(a，b)位于第四象限时，atan2(b，a)取值   -pi/2 ~ 0
%

%中点欧拉法
dheading = diff(path_heading);%差分，size变成length(path_heading) - 1
dheading_pre = [dheading(1);dheading]; %插入一个首元素
dheading_after = [dheading;dheading(end)]; %插入一个尾元素
dheading_final = (dheading_pre + dheading_after) / 2;
%为了防止dheading出现一个2*pi的错误，假设真实的heading较小，用sin(dheading)近似dheading
path_kappa = sin(dheading_final)./ds_final;

== matlab function testEmplanner_cs_referencelinev01/Audi_A8_Sedan_1/decision&planning module/MATLAB Function2 ==
  data: host_match_point_index input; xr output; path_x input; path_y input; paht_heading input; path_kappa input; yr output; thetar output; kappa output
function [xr,yr,thetar,kappa] = fcn(host_match_point_index,path_x,path_y,paht_heading,path_kappa)
index = host_match_point_index(1);
xr = path_x(index + 1);
yr = path_y(index + 1);
thetar = paht_heading(index + 1);
kappa = path_kappa(index + 1);
%#codegen

== matlab function testEmplanner_cs_referencelinev01/Audi_A8_Sedan_1/control module/control main/longitudinal control double PID/MATLAB Function3 ==
  data: kp input; pid_out output; ki input; kd input; err input; err_delay input
function pid_out = fcn(kp,ki,kd,err,err_delay)

persistent integral;
if isempty(integral)
    integral = err * ki *0.01;
    devia = kd*(err - err_delay)/0.01;
    pid_out = kp*err + integral + devia;
else
    integral = integral + err * ki *0.01;
    devia = kd*(err - err_delay)/0.01;
    pid_out = kp*err + integral + devia;
end

== matlab function testEmplanner_cs_referencelinev01/Audi_A8_Sedan_1/control module/control main/lateral control LQR/err_kappa_calculate_module ==
  data: x input; y input; phi input; vx input; vy input; phi_dot input; xr input; yr input; thetar input; kappar input; err output; es output; s_dot output
function [err,es,s_dot] = fcn(x,y,phi,vx,vy,phi_dot,xr,yr,thetar,kappar)
    
    tor=[cos(thetar);sin(thetar)];
    nor=[-sin(thetar);cos(thetar)];
    d_err=[x-xr;y-yr];
    ed=nor'*d_err;
    es=tor'*d_err;
    %projection_point_thetar=thetar(dmin);%apollo
    projection_point_thetar=thetar+kappar*es;
    ed_dot=vy*cos(phi-projection_point_thetar)+vx*sin(phi-projection_point_thetar);
    %%%%%%%%%
    ephi=sin(phi-projection_point_thetar);
    %%%%%%%%%
    ss_dot=vx*cos(phi-projection_point_thetar)-vy*sin(phi-projection_point_thetar);
    s_dot=ss_dot/(1-kappar*ed);
    ephi_dot=phi_dot-kappar*s_dot;
    err=[ed;ed_dot;ephi;ephi_dot];
    
    
    
    
    
    
    
    
    
    
    
    


end

== matlab function testEmplanner_cs_referencelinev01/Audi_A8_Sedan_1/control module/control main/lateral control LQR/feed_forword_control ==
  data: vx input; a input; forword_angle output; b input; m input; cf input; cr input; k input; kr input
function forword_angle = fcn(vx,a,b,m,cf,cr,k,kr)
    forword_angle=kr*(a+b-b*k(3)-(m*vx*vx/(a+b))*((b/cf)+(a/cr)*k(3)-(a/cr)));
end

== matlab function testEmplanner_cs_referencelinev01/Audi_A8_Sedan_1/control module/control main/lateral control LQR/feedback_control+feedforword_control ==
  data: k input; angle output; err input; forword_angle input
function angle = fcn(k,err,forword_angle)

    angle=-k*err+forword_angle;
end

== matlab function testEmplanner_cs_referencelinev01/Audi_A8_Sedan_1/control module/control main/lateral control LQR/calc lqr K ==
  data: k1 input; k output; k2 input; k3 input; k4 input; vx input
function k = fcn(k1,k2,k3,k4,vx)
    if abs(vx) < 0.1 
        k = [0,0,0,0];
    else
        k =[k1,k2,k3,k4];
    end

== matlab function testEmplanner_cs_referencelinev01/Audi_A8_Sedan_1/control module/control main/chassic steering system/MATLAB Function ==
  data: u input; right_steer output; la input; lb input
function right_steer = fcn(u,la,lb)
if abs(u)<1e-2
   right_steer = u;
else
   R =  (la+lb)/tan(u);
   right_steer = atan((la+lb)/(R+1.624/2));
end

== matlab function testEmplanner_cs_referencelinev01/Audi_A8_Sedan_1/control module/control main/lateral control LQR/predict_module ==
  data: x input; pred_x_ctrl output; y input; phi input; vx input; vy input; phi_dot input; ts input; pred_y_ctrl output; pred_yaw_ctrl output; pred_vx_ctrl output; pred_vy_ctrl output; pred_yaw_dot_ctrl output
function [pred_x_ctrl,pred_y_ctrl,pred_yaw_ctrl,pred_vx_ctrl,pred_vy_ctrl,pred_yaw_dot_ctrl] = fcn(x,y,phi,vx,vy,phi_dot,ts)
    pred_x_ctrl=x+vx*ts*cos(phi)-vy*ts*sin(phi);
    pred_y_ctrl=y+vy*ts*cos(phi)+vx*ts*sin(phi);
    pred_yaw_ctrl=phi;
    pred_vx_ctrl=vx;
    pred_vy_ctrl=vy;
    pred_yaw_dot_ctrl=phi_dot;
end

== stateflow chart testEmplanner_cs_referencelinev01/Audi_A8_Sedan_1/Schedule OS ==
  (default) -> (junction 5)
  (junction 5) -> (junction 9) [order 1] : [i>100]
  (junction 5) -> (junction 10) [order 2] : {i = i+1;}
  (junction 9) -> (junction 12) : {
      | do_planning;
      | i = 0;
      | }
  (junction 12) -> (junction 10)
  (junction 10) -> (junction 15)
  (junction 15) -> (junction 17) [order 1] : [j>10]
  (junction 15) -> (junction 21) [order 2] : {j = j+1}
  (junction 17) -> (junction 19) : {
      | do_control;
      | j = 0;
      | }
  (junction 19) -> (junction 21)
  (junction 21) -> (junction 24)
  data: i local =1; j local =1
  events: do_planning output FUNCTION_CALL_EVENT; do_control output FUNCTION_CALL_EVENT

== matlab function testEmplanner_cs_referencelinev01/Audi_A8_Sedan_1/decision&planning module/referenceline provider/MATLAB Function2 ==
  data: host_match_point_index input; referenceline_x_init output; global_path_x input; global_path_y input; referenceline_y_init output
function [referenceline_x_init,referenceline_y_init] = fcn(host_match_point_index,global_path_x,global_path_y)

%该函数将在全局路径上提取referenceline的未平滑的初值
%输入：host_match_point_index 自车的位置在全局路径的匹配点的编号
% global_path_x,global_path_y 全局路径数据

%输出：referenceline_x_init,referenceline_y_init 未平滑的参考线的xy坐标

%由于global_path是每1m取一个点，所以从匹配点I往后取30个点，往前取150个点，一共181个点
%如果前面不够的话，就用后面补，后面不够的话就从前面补，保证总数为181个点。

%索引初始化

start_index = -1;

%判断后面前面的点是否足够多
if host_match_point_index - 30 < 1
	%匹配点前面的数太少了，发生在刚开始
	start_index = 1;
elseif host_match_point_index + 150 > length(global_path_x)
	%匹配点后面的点太少了，发生在结束位置
	start_index = length(global_path_x) - 180;
else 
	%匹配点正常
	start_index = host_match_point_index - 30;
end

%提取reference_line
referenceline_x_init = global_path_x(start_index:start_index+180);%提取，类似于切片
referenceline_y_init = global_path_y(start_index:start_index+180);

== matlab function testEmplanner_cs_referencelinev01/Audi_A8_Sedan_2/PathFollower_Preview_1/LateralController/CTRL REFERENCES/Calculate Lateral Error/eml_find_10k_lateral_error_points ==
  data: pvp input size=2; dist_psvehicle output size=10; TrajOffset_x_y_Y input size=3; ActorOffset_Left_Right input; p0 input size=2; PreviewDistance input size=10; Traj_x parameter; Traj_y parameter; Traj_t parameter; Traj_v parameter; RefreshCounter parameter
function dist_psvehicle  = eml_find_10k_lateral_error_points(pvp,TrajOffset_x_y_Y,ActorOffset_Left_Right,p0,PreviewDistance,Traj_x,Traj_y,Traj_t,Traj_v,RefreshCounter)

dist_psvehicle = emlfcn_find_10k_lateral_error_points(pvp,TrajOffset_x_y_Y,ActorOffset_Left_Right,p0,PreviewDistance,Traj_x,Traj_y,Traj_t,Traj_v,RefreshCounter);

% end function

== matlab function testEmplanner_cs_referencelinev01/Audi_A8_Sedan_1/control module/control main/longitudinal control double PID/MATLAB Function1 ==
  data: u input; throttle output; brake output
function [throttle,brake] = fcn(u)
    if u>=0
        throttle=u;
        brake=0;
    else
        throttle=0;
        brake=-u;
    end

== matlab function testEmplanner_cs_referencelinev01/Audi_A8_Sedan_2/PathFollower_Preview_1/LateralController/CTRL REFERENCES/Find Reference Point (pref0) on Trajectory closest to P0 Point (p0)/eml_find_closest_trajectory_points0 ==
  data: pvp input size=2; Actor_traj_distance output; TrajOffset_x_y_Y input size=3; ActorOffset_Left_Right input; p0 input size=3; Traj_x parameter; Traj_y parameter; Actor_traj_angle output; RefreshCounter parameter
function [Actor_traj_distance,Actor_traj_angle]  = eml_find_closest_trajectory_points0(pvp,TrajOffset_x_y_Y,ActorOffset_Left_Right,p0,Traj_x,Traj_y,RefreshCounter)

[Actor_traj_distance,Actor_traj_angle]  = emlfcn_find_closest_trajectory_points0(pvp,TrajOffset_x_y_Y,ActorOffset_Left_Right,p0,Traj_x,Traj_y,RefreshCounter);

% end function
